simulink model "power_dcdrive_disc"  (Simulink 6.0)
settings: Solver=FixedStepDiscrete  SolverMode=SingleTasking  StartTime=0.0  StopTime=2  FixedStep=Ts  RelTol=1e-3  AbsTol=1e-3
PreLoadFcn:
  | assignin('base','Ts',[10e-6])
undefined symbols (not defined in the file or in its folder): DiscIntNeverNeededParam, find_system, Ts
libraries: powerlib x16, simulink x1, powerlib_extras x1
Description:
  | The 'PreLoadFcn' of power_dcdrive_disc.mdl
  | 
  | automatically sets 'Ts' to 10e-6 in your Workspace.
settings Model: Creator=Hoang Lehuy, Laval University  LastModifiedBy=batserve  ExtModeTrigMode=oneshot  ExtModeArmWhenConnect=off  ExtModeAutoUpdateStatusClock=off
settings DataIOCC: LimitDataPoints=off  SaveFinalState=on  SaveFormat=StructureWithTime  SaveOutput=off  SaveTime=off  SignalLoggingName=sigsOut
settings OptimizationCC: BlockReduction=off  BooleanDataType=off
settings DebuggingCC: CheckExecutionContextPreStartOutputMsg=on  CheckExecutionContextRuntimeOutputMsg=on  SolverPrmCheckMsg=none  UnconnectedInputMsg=none  UnconnectedOutputMsg=none
settings HardwareCC: TargetUnknown=on
settings RTWCC: TemplateMakefile=grt_unix.tmf

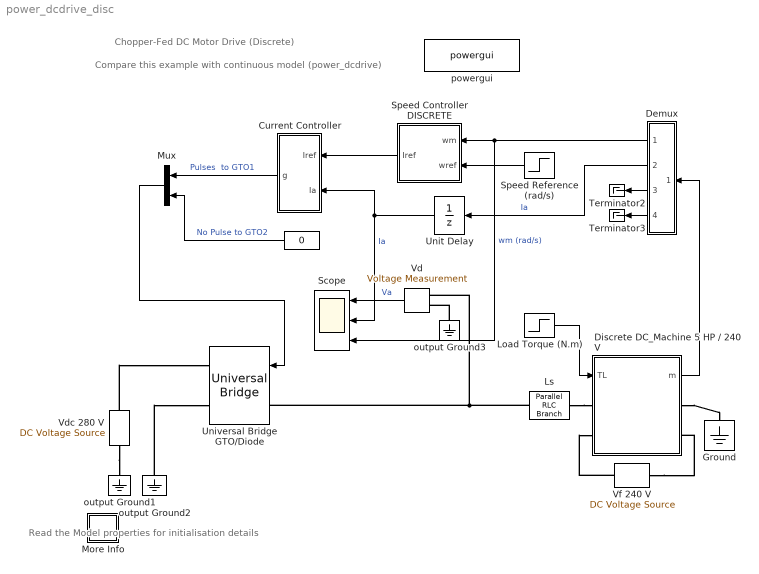
== system power_dcdrive_disc ==
  note: Chopper-Fed DC Motor Drive (Discrete)
  note: Compare this example with continuous model (power_dcdrive)
  note: Read the Model properties
      | for initialisation details
  " " : Constant  Orientation=left  Value=0
  Current Controller : Subsystem  Orientation=left  mask{h=2}
      mask prompts: h "Hysteresis band (A)"
      mask help: Hysteresis Current Controller
      mask Display: plot(0,0,100,100,[45,45],[35,65],[55,55],[35,65],[45,65],[65,65],[35,55],[35,35])
  Demux : Subsystem  Orientation=left
  Discrete DC_Machine 5 HP / 240 V : Subsystem  AncestorBlock=powerlib/Machines/Discrete DC Machine  LoadFcn=find_system(gcs,'FollowLinks', 'on', 'LookUnderMasks', 'all');  mask(Discrete DC machine){RLa=[0.5  0.01], RLf=[240  0], Laf=1.23, J=0.05, Bm=0.02, Tf=0, w0=0, SampleTime=110}
      mask prompts: RLa "Armature resistance and inductance [Ra (ohms) La (H) ]"; RLf "Field resistance and inductance [Rf (ohms) Lf (H) ]"; Laf "Field-armature mutual inductance Laf (H) :"; J "Total inertia J (kg.m^2)"; Bm "Viscous friction coefficient Bm (N.m.s)"; Tf "Coulomb friction torque Tf (N.m)"; w0 "Initial speed (rad/s) :"; SampleTime "Sample Time"
      mask help: This block implements a separately excited DC machine. Access is provided to the field connections so that the machine can be used as a shunt-connected or a series-connected DC machine.
      mask init:
      | Ra=RLa(1); La=RLa(2);
      | 
      | Rf=RLf(1); Lf=RLf(2);
      settings: AttributesFormatString=\n
      mask Help: web(psbhelp)
      mask Display:
      | plot(-80,-80,80,80,[0,9,18,24,29,30,29,24,18,9,0,-9,-18,-24,-29,-30,-29,-24,-18,-9,0],[30,29,24,18,9,0,-9,-18,-24,-29,-30,-29,-24,-18,-9,0,9,18,24,29,30],[-29,-35,-35,-29],[-8,-8,8,8],[29,35,35,29],[-8,-8,8,8],[-35,-55],[0,0],[35,55],[0,0],[-78,-50,-50,-49,-45,-39,-33,-26,-21,-18,-17,-19,-22,-22,-26,-27,-25,-22,-16,-9,-3,2,6,6,4,1,1,-3,-4,-2,2,7,14,20,26,29,30,28,24,24,21,20,21,25,31,37,44,49,50,50,50,78]*.7,[58,58,57.2,49.2,42.8,38.8,38,39.6,44.4,51.6,59.6,67.6,72.4,72.4,65.2,57.2,49.2,42.8,38.8,38,39.6,44.4,51.6,59.6,67.6,72.4,72.4,65.2,57.2,49.2,42.8,38.8,38,39.6,44.4,51.6,59.6,67.6,72.4,72.4,65.2,57.2,49.2,42.8,38.8,38,39.6,44.4,51.6,58,58,58]*.6-85 );
      | 
      | disp('dc')
      | 
      | color('blue');
      | 
      | plot([-50,-10,-10],[50,50,30]);
      | 
      | plot([50,10,10],[50,50,30]);
  Ground : powerlib/Elements/Ground  Orientation=down  PhysicalDomain=powersysdomain  SubClassName=unknown  LeftPortType=p1  RightPortType=p1  LConnTagsString=a
  "Load Torque (N.m) " : Step  Time=1.5  Before=5  After=25  SampleTime=0
  Ls : powerlib/Elements/Parallel RLC Branch  PhysicalDomain=powersysdomain  SubClassName=unknown  LeftPortType=p1  RightPortType=p1  LConnTagsString=a  RConnTagsString=__new0  Resistance=inf  Inductance=10e-03  Capacitance=0  Measurements=None
  More Info : Subsystem
      mask Display: disp('?')
  Mux : Mux  Orientation=left  Inputs=2
  Scope : Scope  NumInputPorts=3
      settings: TickLabels=on  TimeRange=2  YMin=-100~0~-50  YMax=400~40~200  SaveName=var
  Speed Controller DISCRETE : Subsystem  Orientation=left  mask(PI controller){Kp=1.6, Ki=16, Ilim=30, Ts=Ts}
      mask prompts: Kp "Proportional gain (Kp)"; Ki "Integral gain (Ki)"; Ilim "Current limit (A)"; Ts "Sample time (s) :"
      mask help: Proportional-Integral Speed Controller
      mask Display: plot(0,0,100,100,[35,35,65],[70,30,30],[35,65],[45,60])
  Speed Reference (rad/s) : Step  Orientation=left  Time=0.8  Before=120  After=160  SampleTime=0
  Terminator2 : Terminator
  Terminator3 : Terminator
  Unit Delay : UnitDelay  Orientation=left  SampleTime=Ts
  Universal Bridge GTO/Diode : powerlib/Power Electronics/Universal Bridge  Orientation=left  Arms=1  SnubberResistance=10000  SnubberCapacitance=inf  Device=GTO / Diodes  Ron=0.05  Lon=0  ForwardVoltages="[  1  1  ]"  ForwardVoltage=.8  GTOparameters=[ 10e-6 , 20e-6 ]  IGBTparameters=[ 1e-6 , 2e-6 ]  Measurements=None
  Vd : powerlib/Measurements/Voltage Measurement  Tag=PoWeRsYsTeMmEaSuReMeNt  Orientation=left  PhasorSimulation=off  OutputType=Magnitude  PSBequivalent=0
  "Vdc 280 V " : powerlib/Electrical Sources/DC Voltage Source  Description=source block  Orientation=up  Amplitude=280  Measurements=None
      settings: AttributesFormatString=\n
  Vf 240 V : powerlib/Electrical Sources/DC Voltage Source  Description=source block  Orientation=left  Amplitude=240  Measurements=None
      settings: AttributesFormatString=\n
  output Ground1 : powerlib/Elements/Ground  Orientation=down  PhysicalDomain=powersysdomain  SubClassName=unknown  LeftPortType=p1  RightPortType=p1  LConnTagsString=a
  output Ground2 : powerlib/Elements/Ground  Orientation=down  PhysicalDomain=powersysdomain  SubClassName=unknown  LeftPortType=p1  RightPortType=p1  LConnTagsString=a
  output Ground3 : powerlib/Elements/Ground  Orientation=down  PhysicalDomain=powersysdomain  SubClassName=unknown  LeftPortType=p1  RightPortType=p1  LConnTagsString=a
  powergui : powerlib/powergui  Priority=2  Frange=[0:2:500]  Ylog=off  Xlog=on  save=off  variable=ZData  ZoomFFT=on  StartTime=0.0  cycles=1  DisplayStyle=off  fundamental=60  FreqAxis=off  MaxFrequency=1000  frequencyindice=1  frequencyindicesteady=1  RmsSteady=1  display=off  Ts=10e-6  methode=off  frequency=60  echomessages=off
  wires:
  Speed Controller DISCRETE/1(Iref) -> Current Controller/1(Iref)
  Unit Delay/1 -> Current Controller/2(Ia), Scope/2  "Ia"
  Demux/1(wm) -> Speed Controller DISCRETE/1(wm), Scope/3  "wm (rad/s)"
  Demux/2(Ia) -> Unit Delay/1  "Ia"
  Demux/4(Te) -> Terminator3/1
  Demux/3(If) -> Terminator2/1
  Current Controller/1(g) -> Mux/1  "Pulses  to GTO1"
  Speed Reference (rad/s)/1 -> Speed Controller DISCRETE/2(wref)
  " "/1 -> Mux/2  "No Pulse to GTO2"
  Mux/1 -> Universal Bridge GTO/Diode/1
  Vd/1 -> Scope/1  "Va"
  "Load Torque (N.m) "/1 -> Discrete DC_Machine 5 HP / 240 V/1(TL)
  Discrete DC_Machine 5 HP / 240 V/1(m) -> Demux/1(m)
  connections:
  "Vdc 280 V "/RConn1 -- Universal Bridge GTO/Diode/RConn1
  "Vdc 280 V "/LConn1 -- output Ground1/LConn1
  Ls/RConn1 -- Discrete DC_Machine 5 HP / 240 V/LConn1
  Discrete DC_Machine 5 HP / 240 V/RConn1 -- Ground/LConn1
  output Ground2/LConn1 -- Universal Bridge GTO/Diode/RConn2
  Ls/LConn1 -- Universal Bridge GTO/Diode/LConn1 -- Vd/LConn1
  output Ground3/LConn1 -- Vd/LConn2
  Vf 240 V/LConn1 -- Discrete DC_Machine 5 HP / 240 V/RConn2
  Vf 240 V/RConn1 -- Discrete DC_Machine 5 HP / 240 V/LConn2

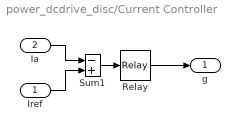
== system power_dcdrive_disc/Current Controller ==
  Iref : Inport  Port=1  LatchInput=off
  Ia : Inport  Port=2  LatchInput=off
  Relay : Relay  OnSwitchValue=h/2  OffSwitchValue=-h/2
  Sum1 : Sum  Inputs=-+  SaturateOnIntegerOverflow=on  InputSameDT=on
  g : Outport  InitialOutput=0
  wires:
  Sum1/1 -> Relay/1
  Relay/1 -> g/1
  Ia/1 -> Sum1/1
  Iref/1 -> Sum1/2

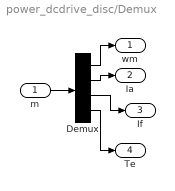
== system power_dcdrive_disc/Demux ==
  m : Inport  Port=1  LatchInput=off
  Demux : Demux
  wm : Outport
  Ia : Outport  Port=2
  If : Outport  Port=3
  Te : Outport  Port=4
  wires:
  Demux/1 -> wm/1
  Demux/2 -> Ia/1
  m/1 -> Demux/1
  Demux/3 -> If/1
  Demux/4 -> Te/1

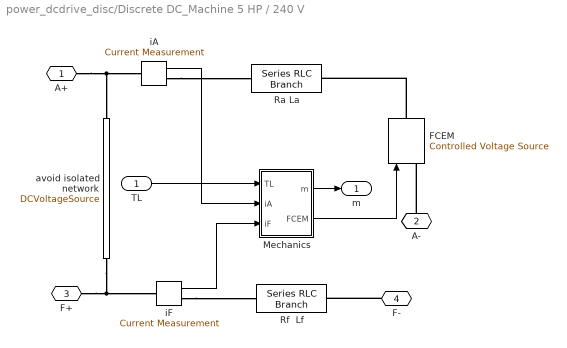
== system power_dcdrive_disc/Discrete DC_Machine 5 HP / 240 V ==
  TL : Inport  Port=1  LatchInput=off
  FCEM : powerlib/Electrical Sources/Controlled Voltage Source  Tag=PoWeRsYsTeMbLoCk  Description=source block  Orientation=up  Initialize=on  Amplitude=0  Phase=0  Frequency=0  Measurements=None
  Mechanics : Subsystem
  Ra La : powerlib/Elements/Series RLC Branch  Tag=PoWeRsYsTeMbLoCk  PhysicalDomain=powersysdomain  SubClassName=unknown  LeftPortType=p1  RightPortType=p1  LConnTagsString=__new0  RConnTagsString=__new0  Resistance=Ra  Inductance=La  Capacitance=inf  Measurements=None
  Rf  Lf : powerlib/Elements/Series RLC Branch  Tag=PoWeRsYsTeMbLoCk  PhysicalDomain=powersysdomain  SubClassName=unknown  LeftPortType=p1  RightPortType=p1  LConnTagsString=__new0  RConnTagsString=__new0  Resistance=Rf  Inductance=Lf  Capacitance=inf  Measurements=None
  avoid isolated network : powerlib/Electrical Sources/DC Voltage Source/DCVoltageSource  Orientation=down  PhysicalDomain=powersysdomain  SubClassName=unknown  LeftPortType=p1  RightPortType=p1  LConnTagsString=a  RConnTagsString=__new0
  iA : powerlib/Measurements/Current Measurement  Tag=PoWeRsYsTeMmEaSuReMeNt  PhasorSimulation=off  OutputType=Magnitude  PSBequivalent=0
  iF : powerlib/Measurements/Current Measurement  Tag=PoWeRsYsTeMmEaSuReMeNt  PhasorSimulation=off  OutputType=Magnitude  PSBequivalent=0
  A+ : PMIOPort  Port=1  Side=Left
  A- : PMIOPort  Orientation=up  Port=2  Side=Right
  F+ : PMIOPort  Port=3  Side=Left
  F- : PMIOPort  Orientation=left  Port=4  Side=Right
  m : Outport
  wires:
  Mechanics/1(m) -> m/1
  TL/1 -> Mechanics/1(TL)
  iF/1 -> Mechanics/3(iF)
  Mechanics/2(FCEM) -> FCEM/1
  iA/1 -> Mechanics/2(iA)
  connections:
  F-/RConn1 -- Rf  Lf/RConn1
  F+/RConn1 -- iF/LConn1 -- avoid isolated network/RConn1
  A-/RConn1 -- FCEM/LConn1
  A+/RConn1 -- iA/LConn1 -- avoid isolated network/LConn1
  iF/RConn1 -- Rf  Lf/LConn1
  iA/RConn1 -- Ra La/LConn1
  FCEM/RConn1 -- Ra La/RConn1

== system power_dcdrive_disc/More Info ==
  note: Chopper-Fed DC Motor Drive (Discrete)
  note: Circuit Description
  note: Demonstration
  note: A DC motor is fed by a DC source through a chopper which consists of GTO thyristor and a free-wheeling diode.
      |
      | The  GTO and diode are simulated with the Universal Bridge block where the number of arms has been set to 1
      | and the  specified power electronic device  is  GTO/Diode. Each switch on the block icon represents a GTO/antiparallel diode pair.
      | Pulses are sent to the top GTO1  only. No pulses are sent to the bottom GTO2.
      | Therefore Diode2 will act as a free wheeling diode.
      |
      | The advantage of using the Universal Bridge block is that  it can be discretized and allows faster simultion speeds
      | than with an individual GTO and Diode. Also, when a purely resistive snubber is used
      | the commutation from GTO to Diode is instantaneous and cleaner wavehapes is obtained for voltage Va
      |
      | The motor drives a mechanical load characterized by inertia J, friction coeficient B, and load torque TL.
      | The motor uses the discrete DC machine provided in the Machines library.
      |
      | The hysteresis current controller compares the sensed current with the reference and generates
      | the trigger signal for the GTO thyristor to force the motor current to follow the reference.
      | The speed control loop uses a proportional-integral controller which produces the reference for the current loop.
      | Current and Voltage Measurement blocks provide signals for visualization purpose.
  note: Start the simulation and observe the motor voltage (Va), current (Ia) and speed  (wm) on the scope.
      | The following observations can be made:
  note: 0< t < 0.8 s: Starting and Steady State Operation
  note: The reference speed  is increased from 120 rad/s to 160 rad/s.
      | The speed controller regulates the speed in approximately 0.25 s, and the average current stabilizes at 6.6 A.
      | During the transient period, current is still maintained at 30 A.
  note: During this period, the load torque is TL = 5.N.m and the motor reaches the reference speed (wref = 120 rad/s) given to the speed controller .
      | The initial values of reference torque and speed are set in the two Step blocks connected to the TL torque input of the motor.
      | Notice that during the motor starting the current is maintained to 30 A, according to the current limit set in the speed regulator.
      | Zoom in the motor current Ia in steady state. Observe the current triangular waveshape varying between 5 A and 7 A,
      | corresponding to the specified hysteresis of 2 A. The commutation frequency is approximately 1.5 kHz.
  note: H. LeHuy (Universite Laval, Quebec) and G. Sybille (Hydro-Quebec)
  note: t = 0.8 s : Reference Speed Step
  note: t = 1.5 s : Load Torque Step
  note: The load torque is suddenly  increased from 5 N.m to 25 N.m.
      | The current increases to 23 A, while the speed is maintained at the 160 rad/s set point.
  note: Note: This example is similar to the continuous version also provided in the Demos library, but discretization allows faster simulation.

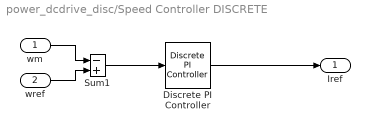
== system power_dcdrive_disc/Speed Controller DISCRETE ==
  wm : Inport  Port=1  LatchInput=off
  wref : Inport  Port=2  LatchInput=off
  Discrete PI Controller : powerlib_extras/Discrete  Control Blocks/Discrete PI Controller  Kp=Kp  Ki=Ki  Par_Limits=[Ilim -Ilim]  Init=0  Ts=Ts
  Sum1 : Sum  Inputs=-+  SaturateOnIntegerOverflow=on  InputSameDT=on
  Iref : Outport  InitialOutput=0
  wires:
  wref/1 -> Sum1/2
  wm/1 -> Sum1/1
  Sum1/1 -> Discrete PI Controller/1
  Discrete PI Controller/1 -> Iref/1

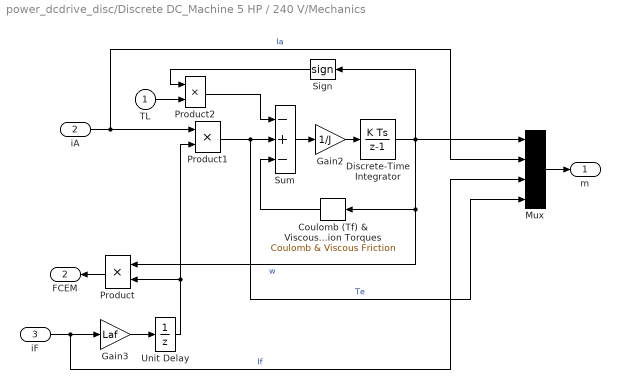
== system power_dcdrive_disc/Discrete DC_Machine 5 HP / 240 V/Mechanics ==
  TL : Inport  Port=1  LatchInput=off
  iA : Inport  Port=2  LatchInput=off
  iF : Inport  Port=3  LatchInput=off
  Coulomb (Tf) & Viscous ( Bm*w)  Friction Torques : simulink/Discontinuities/Coulomb & Viscous Friction  Orientation=left  offset=Tf  gain=Bm
  Discrete-Time Integrator : DiscreteIntegrator  InitialCondition=w0  SampleTime=Ts  ICPrevOutput=DiscIntNeverNeededParam  ICPrevScaledInput=DiscIntNeverNeededParam
  Gain2 : Gain  Gain=1/J  SaturateOnIntegerOverflow=on
  Gain3 : Gain  Gain=Laf  SaturateOnIntegerOverflow=on
  Mux : Mux
  Product : Product  Orientation=left  SaturateOnIntegerOverflow=on  InputSameDT=on
  Product1 : Product  SaturateOnIntegerOverflow=on  InputSameDT=on
  Product2 : Product  SaturateOnIntegerOverflow=on  InputSameDT=on
  Sign : Signum  Orientation=left  ZeroCross=off
  Sum : Sum  Inputs=-+-  SaturateOnIntegerOverflow=on  InputSameDT=on
  Unit Delay : UnitDelay  SampleTime=Ts
  m : Outport
  FCEM : Outport  Orientation=left  Port=2
  wires:
  Coulomb (Tf) & Viscous ( Bm*w)  Friction Torques/1 -> Sum/3
  Product1/1 -> Mux/4, Sum/2  "Te"
  Discrete-Time Integrator/1 -> Sign/1, Mux/1, Product/1, Coulomb (Tf) & Viscous ( Bm*w)  Friction Torques/1  "w"
  Gain2/1 -> Discrete-Time Integrator/1
  Sum/1 -> Gain2/1
  Sign/1 -> Product2/1
  TL/1 -> Product2/2
  Product2/1 -> Sum/1
  iF/1 -> Gain3/1, Mux/3  "If"
  iA/1 -> Product1/1, Mux/2  "Ia"
  Gain3/1 -> Unit Delay/1
  Unit Delay/1 -> Product/2, Product1/2
  Mux/1 -> m/1
  Product/1 -> FCEM/1
